simulink model "Pendulum"  (R2024b)
settings: Solver=VariableStepAuto  StartTime=0.0  StopTime=25  RelTol=1e-3
settings Model: Creator=rares  LastModifiedBy=rares

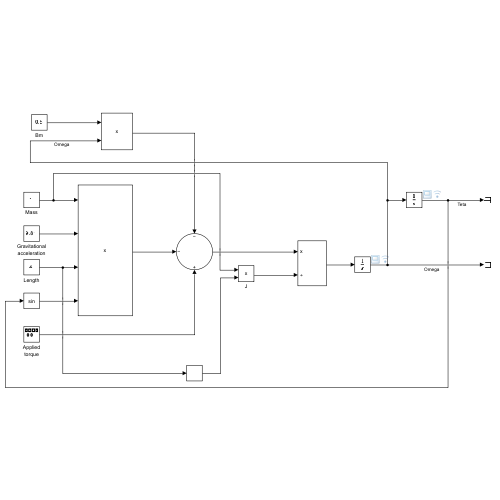
[thumbnail: Simulink's stored preview of the top-level diagram]
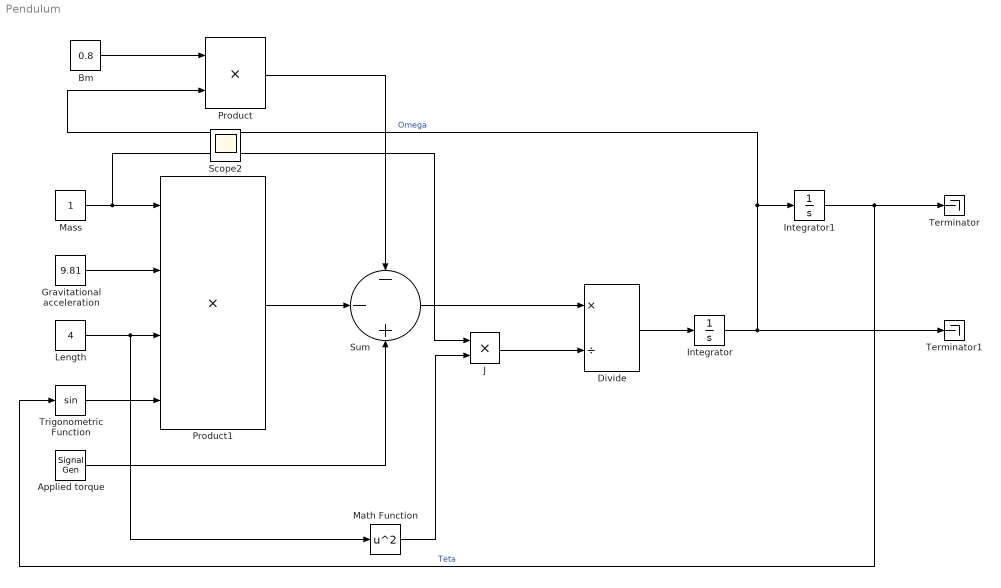
== system Pendulum ==
  Applied torque : SignalGenerator  WaveForm=sawtooth  Frequency=0.1  Units=rad/sec
  Bm : Constant  Value=0.8
  Divide : Product  Inputs=*/
  Gravitational acceleration : Constant  Value=9.81
  Integrator : Integrator
  Integrator1 : Integrator
  J : Product
  Length : Constant  Value=4
  Mass : Constant
  Math Function : Math  Operator=square
  Product : Product
  Product1 : Product  Inputs=4
  Sum : Sum  Inputs=--+
  Terminator : Terminator
  Terminator1 : Terminator
  Trigonometric Function : Trigonometry
  Scope2 : Scope
  wires:
  Bm/1 -> Product/1
  Gravitational acceleration/1 -> Product1/2
  Mass/1 -> Product1/1, J/1
  Length/1 -> Math Function/1, Product1/3
  Product1/1 -> Sum/2
  Product/1 -> Sum/1
  Trigonometric Function/1 -> Product1/4
  Applied torque/1 -> Sum/3
  Sum/1 -> Divide/1
  Math Function/1 -> J/2
  J/1 -> Divide/2
  Divide/1 -> Integrator/1
  Integrator/1 -> Product/2, Integrator1/1, Terminator1/1  "Omega"
  Integrator1/1 -> Terminator/1, Trigonometric Function/1  "Teta"
